simulink model "lotk"  (Simulink 7.6)
settings: Solver=ode45  StartTime=0.0  StopTime=10  MaxStep=0.01  RelTol=1e-3
values from neighbouring files (symbols this model uses):
  e = 0.1    [lotk_script.m]
  e1 = 40    [lotk_script.m]
  e2 = 10    [lotk_script.m]
  K1 = 4000    [lotk_script.m]
  N0 = [25; 10]    [lotk_script.m]
  p = 0.2    [lotk_script.m]
libraries: simulink x1
settings Model: Creator=patrizio  LastModifiedBy=patrizio

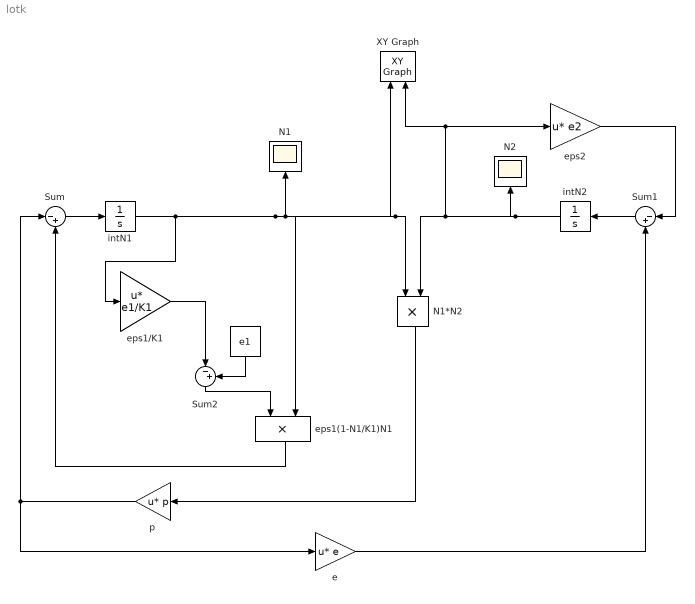
== system lotk ==
  " " : Constant  Value=e1
  N1 : Scope
  N1*N2 : Product  RndMeth=Zero
  N2 : Scope
  Sum : Sum  Inputs=|-+
  Sum1 : Sum  Inputs=|-+
  Sum2 : Sum  Inputs=|-+
  XY Graph : simulink/Sinks/XY Graph  SystemSampleTime=-1  xmin=-20  xmax=20  ymin=-20  ymax=20  st=-1
  e : Gain  Gain=e  Multiplication=Matrix(u*K)
  "eps1(1-N1/K1)N1 " : Product  RndMeth=Zero
  eps1/K1 : Gain  Gain=e1/K1  Multiplication=Matrix(u*K)
  eps2 : Gain  Gain=e2  Multiplication=Matrix(u*K)
  intN1 : Integrator  InitialCondition=N0(1)
  intN2 : Integrator  InitialCondition=N0(2)
  p : Gain  Gain=p  Multiplication=Matrix(u*K)
  wires:
  intN1/1 -> N1*N2/1, XY Graph/1, N1/1, "eps1(1-N1/K1)N1 "/2, eps1/K1/1
  intN2/1 -> N1*N2/2, XY Graph/2, eps2/1, N2/1
  N1*N2/1 -> p/1
  Sum1/1 -> intN2/1
  Sum/1 -> intN1/1
  "eps1(1-N1/K1)N1 "/1 -> Sum/2
  eps1/K1/1 -> Sum2/1
  Sum2/1 -> "eps1(1-N1/K1)N1 "/1
  " "/1 -> Sum2/2
  p/1 -> Sum/1, e/1
  eps2/1 -> Sum1/1
  e/1 -> Sum1/2
